simulink model "driveControl_StateflowChart"  (R2023a)
settings: Solver=VariableStepAuto  StartTime=0.0  StopTime=10.0  RelTol=1e-3
settings Model: Creator=Franz  LastModifiedBy=Franz

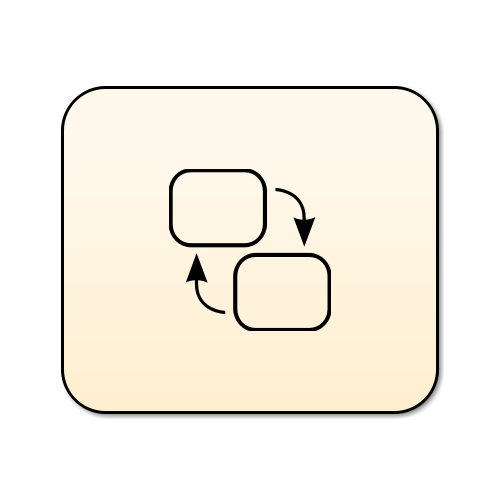
[thumbnail: Simulink's stored preview of the top-level diagram]
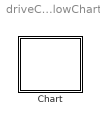
== system driveControl_StateflowChart ==
  Chart : Stateflow chart  TreatAsAtomicUnit=on

== stateflow chart driveControl_StateflowChart/Chart ==
  state chart2
    (default) -> ? [order 4294967295]
    (default) -> ? [order 4294967295]
    (default) -> ? [order 4294967295]
    (default) -> ? [order 4294967295]
  state chart2
  state chart2
    state chartRegion
      state DriveControlComponent
  state chart2
  state chart2
  state chart2
  state chart2
  state chart2
    state chartRegion
      state DriveControlComponent
  state chart2
    state chartRegion
      state DriveControlComponent
  state chart2
    state chartRegion
      state DriveControlComponent
  state chart2
  state communicatorPort
  state communicatorPort
  state communicatorPort
    state WaitForOvertaking
    state WaitforCoordinator
    state Idle
    communicatorPort.WaitforCoordinator -> communicatorPort.Idle [order 1] : denyPermission{communicator_send = 4;}
    communicatorPort.WaitForOvertaking -> communicatorPort.Idle : [communicator_recv == 2]{send(executedOvertaking.overtakingInitPort);}
    communicatorPort.Idle -> communicatorPort.WaitforCoordinator : [communicator_recv==1]{send(OvertakingRequested,overtkingIniPort), coordination_Successfull = true;}
    communicatorPort.WaitforCoordinator -> communicatorPort.WaitForOvertaking [order 2] : grantPermission{communicator_send = 1;}
  state communicatorPort
  state communicatorPort
  state communicatorPort
    state WaitForOvertaking
    state WaitforCoordinator
    state Idle
    communicatorPort.WaitforCoordinator -> communicatorPort.Idle [order 1] : denyPermission{communicator_send = 4;}
    communicatorPort.WaitForOvertaking -> communicatorPort.Idle : [communicator_recv == 2]{send(executedOvertaking.overtakingInitPort);}
    communicatorPort.Idle -> communicatorPort.WaitforCoordinator : [communicator_recv==1]{send(OvertakingRequested,overtkingIniPort), coordination_Successfull = true;}
    communicatorPort.WaitforCoordinator -> communicatorPort.WaitForOvertaking [order 2] : grantPermission{communicator_send = 1;}
  state communicatorPort
    state WaitForOvertaking
    state WaitforCoordinator
    state Idle
    communicatorPort.WaitforCoordinator -> communicatorPort.Idle [order 1] : denyPermission{communicator_send = 4;}
    communicatorPort.WaitForOvertaking -> communicatorPort.Idle : [communicator_recv == 2]{send(executedOvertaking.overtakingInitPort);}
    communicatorPort.Idle -> communicatorPort.WaitforCoordinator : [communicator_recv==1]{send(OvertakingRequested,overtkingIniPort), coordination_Successfull = true;}
    communicatorPort.WaitforCoordinator -> communicatorPort.WaitForOvertaking [order 2] : grantPermission{communicator_send = 1;}
  state communicatorPort
    state WaitForOvertaking
    state WaitforCoordinator
    state Idle
    communicatorPort.WaitforCoordinator -> communicatorPort.Idle [order 1] : denyPermission{communicator_send = 4;}
    communicatorPort.WaitForOvertaking -> communicatorPort.Idle : [communicator_recv == 2]{send(executedOvertaking.overtakingInitPort);}
    communicatorPort.Idle -> communicatorPort.WaitforCoordinator : [communicator_recv==1]{send(OvertakingRequested,overtkingIniPort), coordination_Successfull = true;}
    communicatorPort.WaitforCoordinator -> communicatorPort.WaitForOvertaking [order 2] : grantPermission{communicator_send = 1;}
  state communicatorPort
  state communicatorPort
  state driveControlPort
    state WaitForOvertaking
    state WaitforCoordinator
    state Idle
  state driveControlPort
    state WaitForOvertaking
    state WaitforCoordinator
    state Idle
  state driveControlPort
    state WaitForOvertaking
    state WaitforCoordinator
    state Idle
  state driveControlPort
    state WaitForOvertaking
    state WaitforCoordinator
    state Idle
  state driveControlPort
    state WaitForOvertaking
    state WaitforCoordinator
    state Idle
  state driveControlPort
    state WaitForOvertaking
    state WaitforCoordinator
    state Idle
  state driveControlPort
    state WaitForOvertaking
    state WaitforCoordinator
    state Idle
  state driveControlPort
    state WaitForOvertaking
    state WaitforCoordinator
    state Idle
  state driveControlPort
    state WaitForOvertaking
    state WaitforCoordinator
    state Idle
  state driveControlPort
    state WaitForOvertaking
    state WaitforCoordinator
    state Idle
  state driveControlPort
    state WaitForOvertaking
    state WaitforCoordinator
    state Idle
  state driveControlPort
    state WaitForOvertaking
    state WaitforCoordinator
    state Idle
  state driveControlPort
    state WaitForOvertaking
    state WaitforCoordinator
    state Idle
  state driveControlPort
    state WaitForOvertaking
    state WaitforCoordinator
    state Idle
  state driveControlPort
    state WaitForOvertaking
    state WaitforCoordinator
    state Idle
  state driveControlPort
    state WaitForOvertaking
    state WaitforCoordinator
    state Idle
  state DriveControlComponent
  state DriveControlComponent
  state DriveControlComponent
  state DriveControlComponent
  state DriveControlComponent
  state DriveControlComponent
  state DriveControlComponent
  state DriveControlComponent
  state DriveControlComponent
  state DriveControlComponent
  state DriveControlComponent
  state DriveControlComponent
  state DriveControlComponent
  state chartRegion
  state chartRegion
  state chartRegion
  state chartRegion
  state chartRegion
  state chartRegion
  state chartRegion
  state chartRegion
  state chartRegion
  state chartRegion
  state chartRegion
  state chartRegion
  state chartRegion
  state chart2
  state chart
  state chart2
  state chart
  state chart
  state chart2
    state chartRegion [parallel]
      settings: executionOrder=1
      state DriveControlComponent
  state chart
  state Idle
  state WaitforCoordinator
  state WaitForOvertaking
  (default) -> communicatorPort [order 2]
  (default) -> communicatorPort.Idle [order 3]
  (default) -> communicatorPort [order 4]
  (default) -> communicatorPort.Idle [order 5]
  (default) -> communicatorPort [order 6]
  (default) -> communicatorPort.Idle [order 7]
  (default) -> communicatorPort [order 8]
  (default) -> communicatorPort.Idle [order 9]
  (default) -> communicatorPort [order 10]
  (default) -> driveControlPort.Idle [order 11]
  (default) -> communicatorPort [order 12]
  (default) -> driveControlPort.Idle [order 13]
  (default) -> communicatorPort [order 14]
  (default) -> driveControlPort.Idle [order 15]
  (default) -> communicatorPort [order 16]
  (default) -> driveControlPort.Idle [order 17]
  (default) -> communicatorPort [order 18]
  (default) -> driveControlPort.Idle [order 19]
  (default) -> communicatorPort [order 20]
  (default) -> driveControlPort.Idle [order 21]
  (default) -> DriveControlComponent [order 22]
  (default) -> driveControlPort.Idle [order 23]
  (default) -> chart2.chartRegion.DriveControlComponent [order 24]
  (default) -> driveControlPort.Idle [order 25]
  (default) -> chart2.chartRegion.DriveControlComponent [order 26]
  (default) -> driveControlPort.Idle [order 27]
  (default) -> chart2.chartRegion.DriveControlComponent [order 28]
  (default) -> driveControlPort.Idle [order 29]
  (default) -> chart2.chartRegion.DriveControlComponent [order 30]
  (default) -> driveControlPort.Idle [order 31]
  (default) -> chart2.chartRegion.DriveControlComponent [order 32]
  (default) -> driveControlPort.Idle [order 33]
  driveControlPort.WaitforCoordinator -> driveControlPort.Idle [order 1] : denyPermission{communicator_send = 4;}
  driveControlPort.WaitforCoordinator -> driveControlPort.Idle [order 1] : denyPermission{communicator_send = 4;}
  driveControlPort.WaitforCoordinator -> driveControlPort.Idle [order 1] : denyPermission{communicator_send = 4;}
  driveControlPort.WaitforCoordinator -> driveControlPort.Idle [order 1] : denyPermission{communicator_send = 4;}
  driveControlPort.WaitforCoordinator -> driveControlPort.Idle [order 1] : denyPermission{communicator_send = 4;}
  driveControlPort.WaitforCoordinator -> driveControlPort.Idle [order 1] : denyPermission{communicator_send = 4;}
  driveControlPort.WaitforCoordinator -> driveControlPort.Idle [order 1] : denyPermission{communicator_send = 4;}
  driveControlPort.WaitforCoordinator -> driveControlPort.Idle [order 1] : denyPermission{communicator_send = 4;}
  driveControlPort.WaitforCoordinator -> driveControlPort.Idle [order 1] : denyPermission{communicator_send = 4;}
  driveControlPort.WaitforCoordinator -> driveControlPort.Idle [order 1] : denyPermission{communicator_send = 4;}
  driveControlPort.WaitforCoordinator -> driveControlPort.Idle [order 1] : denyPermission{communicator_send = 4;}
  driveControlPort.WaitforCoordinator -> driveControlPort.Idle [order 1] : denyPermission{communicator_send = 4;}
  driveControlPort.WaitForOvertaking -> driveControlPort.Idle : [communicator_recv == 2]{send(executedOvertaking.overtakingInitPort);}
  driveControlPort.WaitForOvertaking -> driveControlPort.Idle : [communicator_recv == 2]{send(executedOvertaking.overtakingInitPort);}
  driveControlPort.WaitForOvertaking -> driveControlPort.Idle : [communicator_recv == 2]{send(executedOvertaking.overtakingInitPort);}
  driveControlPort.WaitForOvertaking -> driveControlPort.Idle : [communicator_recv == 2]{send(executedOvertaking.overtakingInitPort);}
  driveControlPort.WaitForOvertaking -> driveControlPort.Idle : [communicator_recv == 2]{send(executedOvertaking.overtakingInitPort);}
  driveControlPort.WaitForOvertaking -> driveControlPort.Idle : [communicator_recv == 2]{send(executedOvertaking.overtakingInitPort);}
  driveControlPort.WaitForOvertaking -> driveControlPort.Idle : [communicator_recv == 2]{send(executedOvertaking.overtakingInitPort);}
  driveControlPort.WaitForOvertaking -> driveControlPort.Idle : [communicator_recv == 2]{send(executedOvertaking.overtakingInitPort);}
  driveControlPort.WaitForOvertaking -> driveControlPort.Idle : [communicator_recv == 2]{send(executedOvertaking.overtakingInitPort);}
  driveControlPort.WaitForOvertaking -> driveControlPort.Idle : [communicator_recv == 2]{send(executedOvertaking.overtakingInitPort);}
  driveControlPort.WaitForOvertaking -> driveControlPort.Idle : [communicator_recv == 2]{send(executedOvertaking.overtakingInitPort);}
  driveControlPort.WaitForOvertaking -> driveControlPort.Idle : [communicator_recv == 2]{send(executedOvertaking.overtakingInitPort);}
  driveControlPort.Idle -> driveControlPort.WaitforCoordinator : [communicator_recv==1]{send(OvertakingRequested,overtkingIniPort), coordination_Successfull = true;}
  driveControlPort.Idle -> driveControlPort.WaitforCoordinator : [communicator_recv==1]{send(OvertakingRequested,overtkingIniPort), coordination_Successfull = true;}
  driveControlPort.Idle -> driveControlPort.WaitforCoordinator : [communicator_recv==1]{send(OvertakingRequested,overtkingIniPort), coordination_Successfull = true;}
  driveControlPort.Idle -> driveControlPort.WaitforCoordinator : [communicator_recv==1]{send(OvertakingRequested,overtkingIniPort), coordination_Successfull = true;}
  driveControlPort.Idle -> driveControlPort.WaitforCoordinator : [communicator_recv==1]{send(OvertakingRequested,overtkingIniPort), coordination_Successfull = true;}
  driveControlPort.Idle -> driveControlPort.WaitforCoordinator : [communicator_recv==1]{send(OvertakingRequested,overtkingIniPort), coordination_Successfull = true;}
  driveControlPort.Idle -> driveControlPort.WaitforCoordinator : [communicator_recv==1]{send(OvertakingRequested,overtkingIniPort), coordination_Successfull = true;}
  driveControlPort.Idle -> driveControlPort.WaitforCoordinator : [communicator_recv==1]{send(OvertakingRequested,overtkingIniPort), coordination_Successfull = true;}
  driveControlPort.Idle -> driveControlPort.WaitforCoordinator : [communicator_recv==1]{send(OvertakingRequested,overtkingIniPort), coordination_Successfull = true;}
  driveControlPort.Idle -> driveControlPort.WaitforCoordinator : [communicator_recv==1]{send(OvertakingRequested,overtkingIniPort), coordination_Successfull = true;}
  driveControlPort.Idle -> driveControlPort.WaitforCoordinator : [communicator_recv==1]{send(OvertakingRequested,overtkingIniPort), coordination_Successfull = true;}
  driveControlPort.Idle -> driveControlPort.WaitforCoordinator : [communicator_recv==1]{send(OvertakingRequested,overtkingIniPort), coordination_Successfull = true;}
  driveControlPort.WaitforCoordinator -> driveControlPort.WaitForOvertaking [order 2] : grantPermission{communicator_send = 1;}
  driveControlPort.WaitforCoordinator -> driveControlPort.WaitForOvertaking [order 2] : grantPermission{communicator_send = 1;}
  driveControlPort.WaitforCoordinator -> driveControlPort.WaitForOvertaking [order 2] : grantPermission{communicator_send = 1;}
  driveControlPort.WaitforCoordinator -> driveControlPort.WaitForOvertaking [order 2] : grantPermission{communicator_send = 1;}
  driveControlPort.WaitforCoordinator -> driveControlPort.WaitForOvertaking [order 2] : grantPermission{communicator_send = 1;}
  driveControlPort.WaitforCoordinator -> driveControlPort.WaitForOvertaking [order 2] : grantPermission{communicator_send = 1;}
  driveControlPort.WaitforCoordinator -> driveControlPort.WaitForOvertaking [order 2] : grantPermission{communicator_send = 1;}
  driveControlPort.WaitforCoordinator -> driveControlPort.WaitForOvertaking [order 2] : grantPermission{communicator_send = 1;}
  driveControlPort.WaitforCoordinator -> driveControlPort.WaitForOvertaking [order 2] : grantPermission{communicator_send = 1;}
  driveControlPort.WaitforCoordinator -> driveControlPort.WaitForOvertaking [order 2] : grantPermission{communicator_send = 1;}
  driveControlPort.WaitforCoordinator -> driveControlPort.WaitForOvertaking [order 2] : grantPermission{communicator_send = 1;}
  driveControlPort.WaitforCoordinator -> driveControlPort.WaitForOvertaking [order 2] : grantPermission{communicator_send = 1;}
  WaitforCoordinator -> Idle [order 1] : denyPermission{communicator_send = 4;}
  (default) -> Idle [order 1]
  WaitforCoordinator -> WaitForOvertaking [order 2] : grantPermission{communicator_send = 1;}
  Idle -> WaitforCoordinator : [communicator_recv==1]{send(OvertakingRequested,overtkingIniPort), coordination_Successfull = true;}
  WaitForOvertaking -> Idle : [communicator_recv == 2]{send(executedOvertaking.overtakingInitPort);}
